simulink model "zadanie2"  (R2025a)
settings: Solver=VariableStepAuto  StartTime=0.0  StopTime=20  RelTol=1e-3
values from neighbouring files (symbols this model uses):
  L = 3    [cvico3_zlepsenie.m]
  LD = 2    [cvico3_zlepsenie.m]
  xRef = xRef2s    [cvico3_zlepsenie.m]    (also in setUpModel.m = refPose(:,1))
  yRef = yRef2s    [cvico3_zlepsenie.m]    (also in setUpModel.m = -refPose(:,2))
libraries: robotalgslib x1, autolibshared x1
settings Model: Creator=ASUS  LastModifiedBy=ASUS

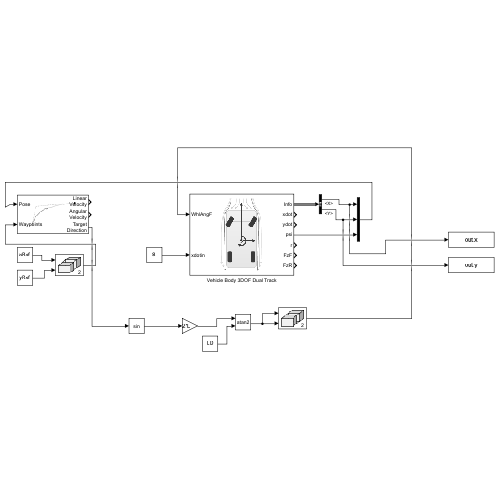
[thumbnail: Simulink's stored preview of the top-level diagram]
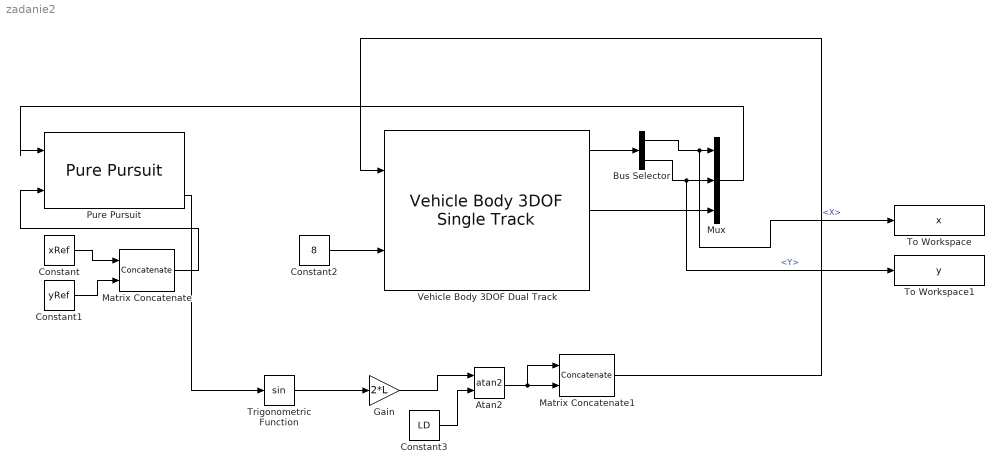
== system zadanie2 ==
  Atan2 : Trigonometry  Operator=atan2
  Bus Selector : BusSelector  OutputSignals=InertFrm.Cg.Disp.X,InertFrm.Cg.Disp.Y
  Constant : Constant  Value=xRef
  Constant1 : Constant  Value=yRef
  Constant2 : Constant  Value=8
  Constant3 : Constant  Value=LD
  Gain : Gain  Gain=2*L
  Matrix Concatenate : Concatenate  Mode=Multidimensional array  ConcatenateDimension=2
  Matrix Concatenate1 : Concatenate  Mode=Multidimensional array  ConcatenateDimension=2
  Mux : Mux  Inputs=3
  Pure Pursuit : robotalgslib/Pure Pursuit  DesiredLinearVelocityPort=off  DesiredLinearVelocity=0.1  MaxAngularVelocity=1.0  LookaheadDistancePort=off  LookaheadDistance=LD  TargetDirPort=on  SimulateUsing=Code generation
      settings: LibrarySourceBlock=navlib/Control Algorithms/Pure Pursuit
  To Workspace : ToWorkspace  VariableName=x  SampleTime=0.1
  To Workspace1 : ToWorkspace  VariableName=y  SampleTime=0.1
  Trigonometric Function : Trigonometry
  Vehicle Body 3DOF Dual Track : autolibshared/Vehicle Body 3DOF Single Track  trackMode=Dual  inputMode=External longitudinal velocity  frontSteerMode=on  rearSteerMode=off  windMode=off  muMode=off  extFMode=off  extMMode=off  htchFMode=off  htchMMode=off  extXo=off  extpsio=off  extxdoto=off  extro=off  extYo=off  extTamb=off  extydoto=off  aMode=2  NF=2  NR=2  m=2000  a=1.4  b=1.6  h=0.35  dh=1  hh=0.2  X_o=x0  xdot_o=0  CalphaMode=off  sigmaMode=on  d=0  hl=0  w=[1.4,1.4]  Cy_f=12e3  Cy_r=11e3  sigma_f=.1  sigma_r=.1  alpha_f_brk=[-.1 .1]  Cy_f_data=[-9e3 9e3]  alpha_r_brk=[-.1 .1]  Cy_r_data=[-9e3 9e3]  Y_o=y0  ydot_o=0  Izz=4000  psi_o=psi0  r_o=0  Af=2  Cd=.3  Cl=.1  Cpm=.1  beta_w=[0 0.01:0.01:0.3]  Cs=[0:0.03:0.9]  Cym=[0 1e-6:0.01:0.3]  Pabs=101325  Tair=273  g=9.81  mu=1  xdot_tol=.01  Fznom=5000  Fxtire_sat=7e4  Fytire_sat=7e4  longOff=0  latOff=0  vertOff=0  wrapAng=off
      settings: LibrarySourceBlock=vehdynlibeom/Vehicle Body 3DOF Dual Track
  wires:
  Vehicle Body 3DOF Dual Track/1 -> Bus Selector/1
  Bus Selector/1 -> To Workspace/1, Mux/1  "<X>"
  Bus Selector/2 -> To Workspace1/1, Mux/2  "<Y>"
  Vehicle Body 3DOF Dual Track/4 -> Mux/3
  Mux/1 -> Pure Pursuit/1
  Constant/1 -> Matrix Concatenate/1
  Constant1/1 -> Matrix Concatenate/2
  Matrix Concatenate/1 -> Pure Pursuit/2
  Constant2/1 -> Vehicle Body 3DOF Dual Track/2
  Trigonometric Function/1 -> Gain/1
  Gain/1 -> Atan2/1
  Constant3/1 -> Atan2/2
  Atan2/1 -> Matrix Concatenate1/1, Matrix Concatenate1/2
  Matrix Concatenate1/1 -> Vehicle Body 3DOF Dual Track/1
  Pure Pursuit/3 -> Trigonometric Function/1
